simulink model "computed_torques_sim"  (R2019b)
settings: Solver=VariableStepAuto  StartTime=0.0  StopTime=10  MaxStep=1e-2  RelTol=1e-3
model workspace: external: MATLAB File /Users/simonlangbak/Desktop/CrustCrawlerModel/crustcrawler_DataFile.m (data not in the file)
undefined symbols (not defined in the file or in its folder): smiData, X, Y, Z
libraries: sm_lib x100, nesl_utility x10
(part 2 of 3)

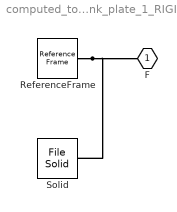
== system computed_torques_sim/Link 5/Link_plate_1_RIGID ==
  ReferenceFrame : sm_lib/Frames and Transforms/Reference Frame
  Solid : sm_lib/Body Elements/File Solid  ExtGeomFileName=Link-plate_Default_sldprt.STEP  UnitType=FromFile  ExtGeomFileUnits=m  StepReaderType=HEX  ExportEntireGeometry=off  InertiaType=Custom  Mass=smiData.Solid(7).mass  MassUnits=kg  CenterOfMass=smiData.Solid(7).CoM  CenterOfMassUnits=mm  MomentsOfInertia=smiData.Solid(7).MoI  MomentsOfInertiaUnits=kg*mm^2  ProductsOfInertia=smiData.Solid(7).PoI  ProductsOfInertiaUnits=kg*mm^2  BasedOnType=DensityFromFile  Density=1000  DensityUnits=kg/m^3  DoExposeReferenceFrame=on  SerializedFrames=<Frames/>  GraphicType=FromGeometry  MarkerShape=Sphere  MarkerSize=10  GraphicVisPropType=SimpleVisualProperties  GraphicDiffuseColor=smiData.Solid(7).color  GraphicSpecularColor=[0.5 0.5 0.5 1.0]  GraphicAmbientColor=[0.15 0.15 0.15 1.0]  GraphicEmissiveColor=[0.0 0.0 0.0 1.0]  GraphicShininess=75  GraphicOpacity=smiData.Solid(7).opacity
  F : PMIOPort  Side=Left
  connections:
  Solid/RConn1 -- ReferenceFrame/RConn1 -- F/RConn1

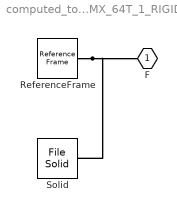
== system computed_torques_sim/Link 5/MX_64T_1_RIGID ==
  ReferenceFrame : sm_lib/Frames and Transforms/Reference Frame
  Solid : sm_lib/Body Elements/File Solid  ExtGeomFileName=MX-64T_Default_sldprt.STEP  UnitType=FromFile  ExtGeomFileUnits=m  StepReaderType=HEX  ExportEntireGeometry=off  InertiaType=Custom  Mass=smiData.Solid(14).mass  MassUnits=kg  CenterOfMass=smiData.Solid(14).CoM  CenterOfMassUnits=mm  MomentsOfInertia=smiData.Solid(14).MoI  MomentsOfInertiaUnits=kg*mm^2  ProductsOfInertia=smiData.Solid(14).PoI  ProductsOfInertiaUnits=kg*mm^2  BasedOnType=DensityFromFile  Density=1000  DensityUnits=kg/m^3  DoExposeReferenceFrame=on  SerializedFrames=<Frames/>  GraphicType=FromGeometry  MarkerShape=Sphere  MarkerSize=10  GraphicVisPropType=SimpleVisualProperties  GraphicDiffuseColor=smiData.Solid(14).color  GraphicSpecularColor=[0.5 0.5 0.5 1.0]  GraphicAmbientColor=[0.15 0.15 0.15 1.0]  GraphicEmissiveColor=[0.0 0.0 0.0 1.0]  GraphicShininess=75  GraphicOpacity=smiData.Solid(14).opacity
  F : PMIOPort  Side=Left
  connections:
  Solid/RConn1 -- ReferenceFrame/RConn1 -- F/RConn1

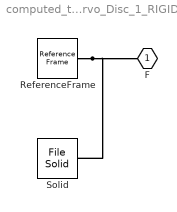
== system computed_torques_sim/Link 5/Servo_Disc_1_RIGID ==
  ReferenceFrame : sm_lib/Frames and Transforms/Reference Frame
  Solid : sm_lib/Body Elements/File Solid  ExtGeomFileName=Servo-Disc_Default_sldprt.STEP  UnitType=FromFile  ExtGeomFileUnits=m  StepReaderType=HEX  ExportEntireGeometry=off  InertiaType=Custom  Mass=smiData.Solid(3).mass  MassUnits=kg  CenterOfMass=smiData.Solid(3).CoM  CenterOfMassUnits=mm  MomentsOfInertia=smiData.Solid(3).MoI  MomentsOfInertiaUnits=kg*mm^2  ProductsOfInertia=smiData.Solid(3).PoI  ProductsOfInertiaUnits=kg*mm^2  BasedOnType=DensityFromFile  Density=1000  DensityUnits=kg/m^3  DoExposeReferenceFrame=on  SerializedFrames=<Frames/>  GraphicType=FromGeometry  MarkerShape=Sphere  MarkerSize=10  GraphicVisPropType=SimpleVisualProperties  GraphicDiffuseColor=smiData.Solid(3).color  GraphicSpecularColor=[0.5 0.5 0.5 1.0]  GraphicAmbientColor=[0.15 0.15 0.15 1.0]  GraphicEmissiveColor=[0.0 0.0 0.0 1.0]  GraphicShininess=75  GraphicOpacity=smiData.Solid(3).opacity
  F : PMIOPort  Side=Left
  connections:
  Solid/RConn1 -- ReferenceFrame/RConn1 -- F/RConn1

== system computed_torques_sim/Link 5/Servo_Disc_2_RIGID ==
  ReferenceFrame : sm_lib/Frames and Transforms/Reference Frame
  Solid : sm_lib/Body Elements/File Solid  ExtGeomFileName=Servo-Disc_Default_sldprt.STEP  UnitType=FromFile  ExtGeomFileUnits=m  StepReaderType=HEX  ExportEntireGeometry=off  InertiaType=Custom  Mass=smiData.Solid(3).mass  MassUnits=kg  CenterOfMass=smiData.Solid(3).CoM  CenterOfMassUnits=mm  MomentsOfInertia=smiData.Solid(3).MoI  MomentsOfInertiaUnits=kg*mm^2  ProductsOfInertia=smiData.Solid(3).PoI  ProductsOfInertiaUnits=kg*mm^2  BasedOnType=DensityFromFile  Density=1000  DensityUnits=kg/m^3  DoExposeReferenceFrame=on  SerializedFrames=<Frames/>  GraphicType=FromGeometry  MarkerShape=Sphere  MarkerSize=10  GraphicVisPropType=SimpleVisualProperties  GraphicDiffuseColor=smiData.Solid(3).color  GraphicSpecularColor=[0.5 0.5 0.5 1.0]  GraphicAmbientColor=[0.15 0.15 0.15 1.0]  GraphicEmissiveColor=[0.0 0.0 0.0 1.0]  GraphicShininess=75  GraphicOpacity=smiData.Solid(3).opacity
  F : PMIOPort  Side=Left
  connections:
  Solid/RConn1 -- ReferenceFrame/RConn1 -- F/RConn1

== system computed_torques_sim/Link 5/Servo_disc_link_MX_106T_1_RIGID ==
  ReferenceFrame : sm_lib/Frames and Transforms/Reference Frame
  Solid : sm_lib/Body Elements/File Solid  ExtGeomFileName=Servo-disc-link_MX-106T_Default_sldprt.STEP  UnitType=FromFile  ExtGeomFileUnits=m  StepReaderType=HEX  ExportEntireGeometry=off  InertiaType=Custom  Mass=smiData.Solid(16).mass  MassUnits=kg  CenterOfMass=smiData.Solid(16).CoM  CenterOfMassUnits=mm  MomentsOfInertia=smiData.Solid(16).MoI  MomentsOfInertiaUnits=kg*mm^2  ProductsOfInertia=smiData.Solid(16).PoI  ProductsOfInertiaUnits=kg*mm^2  BasedOnType=DensityFromFile  Density=1000  DensityUnits=kg/m^3  DoExposeReferenceFrame=on  SerializedFrames=<Frames/>  GraphicType=FromGeometry  MarkerShape=Sphere  MarkerSize=10  GraphicVisPropType=SimpleVisualProperties  GraphicDiffuseColor=smiData.Solid(16).color  GraphicSpecularColor=[0.5 0.5 0.5 1.0]  GraphicAmbientColor=[0.15 0.15 0.15 1.0]  GraphicEmissiveColor=[0.0 0.0 0.0 1.0]  GraphicShininess=75  GraphicOpacity=smiData.Solid(16).opacity
  F : PMIOPort  Side=Left
  connections:
  Solid/RConn1 -- ReferenceFrame/RConn1 -- F/RConn1

== system computed_torques_sim/Link 5/Servo_link_link_MX_64T_1_RIGID ==
  ReferenceFrame : sm_lib/Frames and Transforms/Reference Frame
  Solid : sm_lib/Body Elements/File Solid  ExtGeomFileName=Servo-link-link_MX-64T_Default_sldprt.STEP  UnitType=FromFile  ExtGeomFileUnits=m  StepReaderType=HEX  ExportEntireGeometry=off  InertiaType=Custom  Mass=smiData.Solid(13).mass  MassUnits=kg  CenterOfMass=smiData.Solid(13).CoM  CenterOfMassUnits=mm  MomentsOfInertia=smiData.Solid(13).MoI  MomentsOfInertiaUnits=kg*mm^2  ProductsOfInertia=smiData.Solid(13).PoI  ProductsOfInertiaUnits=kg*mm^2  BasedOnType=DensityFromFile  Density=1000  DensityUnits=kg/m^3  DoExposeReferenceFrame=on  SerializedFrames=<Frames/>  GraphicType=FromGeometry  MarkerShape=Sphere  MarkerSize=10  GraphicVisPropType=SimpleVisualProperties  GraphicDiffuseColor=smiData.Solid(13).color  GraphicSpecularColor=[0.5 0.5 0.5 1.0]  GraphicAmbientColor=[0.15 0.15 0.15 1.0]  GraphicEmissiveColor=[0.0 0.0 0.0 1.0]  GraphicShininess=75  GraphicOpacity=smiData.Solid(13).opacity
  F : PMIOPort  Side=Left
  connections:
  Solid/RConn1 -- ReferenceFrame/RConn1 -- F/RConn1

== system computed_torques_sim/Link 6/Finger_1_RIGID ==
  ReferenceFrame : sm_lib/Frames and Transforms/Reference Frame
  Solid : sm_lib/Body Elements/File Solid  ExtGeomFileName=Finger_Default_sldprt.STEP  UnitType=FromFile  ExtGeomFileUnits=m  StepReaderType=HEX  ExportEntireGeometry=off  InertiaType=Custom  Mass=smiData.Solid(4).mass  MassUnits=kg  CenterOfMass=smiData.Solid(4).CoM  CenterOfMassUnits=mm  MomentsOfInertia=smiData.Solid(4).MoI  MomentsOfInertiaUnits=kg*mm^2  ProductsOfInertia=smiData.Solid(4).PoI  ProductsOfInertiaUnits=kg*mm^2  BasedOnType=DensityFromFile  Density=1000  DensityUnits=kg/m^3  DoExposeReferenceFrame=on  SerializedFrames=<Frames/>  GraphicType=FromGeometry  MarkerShape=Sphere  MarkerSize=10  GraphicVisPropType=SimpleVisualProperties  GraphicDiffuseColor=smiData.Solid(4).color  GraphicSpecularColor=[0.5 0.5 0.5 1.0]  GraphicAmbientColor=[0.15 0.15 0.15 1.0]  GraphicEmissiveColor=[0.0 0.0 0.0 1.0]  GraphicShininess=75  GraphicOpacity=smiData.Solid(4).opacity
  F : PMIOPort  Side=Left
  connections:
  Solid/RConn1 -- ReferenceFrame/RConn1 -- F/RConn1

== system computed_torques_sim/Link 6/Finger_2_RIGID ==
  ReferenceFrame : sm_lib/Frames and Transforms/Reference Frame
  Solid : sm_lib/Body Elements/File Solid  ExtGeomFileName=Finger_Default_sldprt.STEP  UnitType=FromFile  ExtGeomFileUnits=m  StepReaderType=HEX  ExportEntireGeometry=off  InertiaType=Custom  Mass=smiData.Solid(4).mass  MassUnits=kg  CenterOfMass=smiData.Solid(4).CoM  CenterOfMassUnits=mm  MomentsOfInertia=smiData.Solid(4).MoI  MomentsOfInertiaUnits=kg*mm^2  ProductsOfInertia=smiData.Solid(4).PoI  ProductsOfInertiaUnits=kg*mm^2  BasedOnType=DensityFromFile  Density=1000  DensityUnits=kg/m^3  DoExposeReferenceFrame=on  SerializedFrames=<Frames/>  GraphicType=FromGeometry  MarkerShape=Sphere  MarkerSize=10  GraphicVisPropType=SimpleVisualProperties  GraphicDiffuseColor=smiData.Solid(4).color  GraphicSpecularColor=[0.5 0.5 0.5 1.0]  GraphicAmbientColor=[0.15 0.15 0.15 1.0]  GraphicEmissiveColor=[0.0 0.0 0.0 1.0]  GraphicShininess=75  GraphicOpacity=smiData.Solid(4).opacity
  F : PMIOPort  Side=Left
  connections:
  Solid/RConn1 -- ReferenceFrame/RConn1 -- F/RConn1

== system computed_torques_sim/Link 6/Link_2_1_RIGID ==
  ReferenceFrame : sm_lib/Frames and Transforms/Reference Frame
  Solid : sm_lib/Body Elements/File Solid  ExtGeomFileName=Link-2_Default_sldprt.STEP  UnitType=FromFile  ExtGeomFileUnits=m  StepReaderType=HEX  ExportEntireGeometry=off  InertiaType=Custom  Mass=smiData.Solid(8).mass  MassUnits=kg  CenterOfMass=smiData.Solid(8).CoM  CenterOfMassUnits=mm  MomentsOfInertia=smiData.Solid(8).MoI  MomentsOfInertiaUnits=kg*mm^2  ProductsOfInertia=smiData.Solid(8).PoI  ProductsOfInertiaUnits=kg*mm^2  BasedOnType=DensityFromFile  Density=1000  DensityUnits=kg/m^3  DoExposeReferenceFrame=on  SerializedFrames=<Frames/>  GraphicType=FromGeometry  MarkerShape=Sphere  MarkerSize=10  GraphicVisPropType=SimpleVisualProperties  GraphicDiffuseColor=smiData.Solid(8).color  GraphicSpecularColor=[0.5 0.5 0.5 1.0]  GraphicAmbientColor=[0.15 0.15 0.15 1.0]  GraphicEmissiveColor=[0.0 0.0 0.0 1.0]  GraphicShininess=75  GraphicOpacity=smiData.Solid(8).opacity
  F : PMIOPort  Side=Left
  connections:
  Solid/RConn1 -- ReferenceFrame/RConn1 -- F/RConn1

== system computed_torques_sim/Link 6/Link_plate_1_RIGID ==
  ReferenceFrame : sm_lib/Frames and Transforms/Reference Frame
  Solid : sm_lib/Body Elements/File Solid  ExtGeomFileName=Link-plate_Default_sldprt.STEP  UnitType=FromFile  ExtGeomFileUnits=m  StepReaderType=HEX  ExportEntireGeometry=off  InertiaType=Custom  Mass=smiData.Solid(7).mass  MassUnits=kg  CenterOfMass=smiData.Solid(7).CoM  CenterOfMassUnits=mm  MomentsOfInertia=smiData.Solid(7).MoI  MomentsOfInertiaUnits=kg*mm^2  ProductsOfInertia=smiData.Solid(7).PoI  ProductsOfInertiaUnits=kg*mm^2  BasedOnType=DensityFromFile  Density=1000  DensityUnits=kg/m^3  DoExposeReferenceFrame=on  SerializedFrames=<Frames/>  GraphicType=FromGeometry  MarkerShape=Sphere  MarkerSize=10  GraphicVisPropType=SimpleVisualProperties  GraphicDiffuseColor=smiData.Solid(7).color  GraphicSpecularColor=[0.5 0.5 0.5 1.0]  GraphicAmbientColor=[0.15 0.15 0.15 1.0]  GraphicEmissiveColor=[0.0 0.0 0.0 1.0]  GraphicShininess=75  GraphicOpacity=smiData.Solid(7).opacity
  F : PMIOPort  Side=Left
  connections:
  Solid/RConn1 -- ReferenceFrame/RConn1 -- F/RConn1

== system computed_torques_sim/Link 6/MX_28T_1_RIGID ==
  ReferenceFrame : sm_lib/Frames and Transforms/Reference Frame
  Solid : sm_lib/Body Elements/File Solid  ExtGeomFileName=MX-28T_Default_sldprt.STEP  UnitType=FromFile  ExtGeomFileUnits=m  StepReaderType=HEX  ExportEntireGeometry=off  InertiaType=Custom  Mass=smiData.Solid(5).mass  MassUnits=kg  CenterOfMass=smiData.Solid(5).CoM  CenterOfMassUnits=mm  MomentsOfInertia=smiData.Solid(5).MoI  MomentsOfInertiaUnits=kg*mm^2  ProductsOfInertia=smiData.Solid(5).PoI  ProductsOfInertiaUnits=kg*mm^2  BasedOnType=DensityFromFile  Density=1000  DensityUnits=kg/m^3  DoExposeReferenceFrame=on  SerializedFrames=<Frames/>  GraphicType=FromGeometry  MarkerShape=Sphere  MarkerSize=10  GraphicVisPropType=SimpleVisualProperties  GraphicDiffuseColor=smiData.Solid(5).color  GraphicSpecularColor=[0.5 0.5 0.5 1.0]  GraphicAmbientColor=[0.15 0.15 0.15 1.0]  GraphicEmissiveColor=[0.0 0.0 0.0 1.0]  GraphicShininess=75  GraphicOpacity=smiData.Solid(5).opacity
  F : PMIOPort  Side=Left
  connections:
  Solid/RConn1 -- ReferenceFrame/RConn1 -- F/RConn1

== system computed_torques_sim/Link 6/MX_28T_2_RIGID ==
  ReferenceFrame : sm_lib/Frames and Transforms/Reference Frame
  Solid : sm_lib/Body Elements/File Solid  ExtGeomFileName=MX-28T_Default_sldprt.STEP  UnitType=FromFile  ExtGeomFileUnits=m  StepReaderType=HEX  ExportEntireGeometry=off  InertiaType=Custom  Mass=smiData.Solid(5).mass  MassUnits=kg  CenterOfMass=smiData.Solid(5).CoM  CenterOfMassUnits=mm  MomentsOfInertia=smiData.Solid(5).MoI  MomentsOfInertiaUnits=kg*mm^2  ProductsOfInertia=smiData.Solid(5).PoI  ProductsOfInertiaUnits=kg*mm^2  BasedOnType=DensityFromFile  Density=1000  DensityUnits=kg/m^3  DoExposeReferenceFrame=on  SerializedFrames=<Frames/>  GraphicType=FromGeometry  MarkerShape=Sphere  MarkerSize=10  GraphicVisPropType=SimpleVisualProperties  GraphicDiffuseColor=smiData.Solid(5).color  GraphicSpecularColor=[0.5 0.5 0.5 1.0]  GraphicAmbientColor=[0.15 0.15 0.15 1.0]  GraphicEmissiveColor=[0.0 0.0 0.0 1.0]  GraphicShininess=75  GraphicOpacity=smiData.Solid(5).opacity
  F : PMIOPort  Side=Left
  connections:
  Solid/RConn1 -- ReferenceFrame/RConn1 -- F/RConn1

== system computed_torques_sim/Link 6/MX_28T_Link_1_RIGID ==
  ReferenceFrame : sm_lib/Frames and Transforms/Reference Frame
  Solid : sm_lib/Body Elements/File Solid  ExtGeomFileName=MX-28T-Link_Default_sldprt.STEP  UnitType=FromFile  ExtGeomFileUnits=m  StepReaderType=HEX  ExportEntireGeometry=off  InertiaType=Custom  Mass=smiData.Solid(9).mass  MassUnits=kg  CenterOfMass=smiData.Solid(9).CoM  CenterOfMassUnits=mm  MomentsOfInertia=smiData.Solid(9).MoI  MomentsOfInertiaUnits=kg*mm^2  ProductsOfInertia=smiData.Solid(9).PoI  ProductsOfInertiaUnits=kg*mm^2  BasedOnType=DensityFromFile  Density=1000  DensityUnits=kg/m^3  DoExposeReferenceFrame=on  SerializedFrames=<Frames/>  GraphicType=FromGeometry  MarkerShape=Sphere  MarkerSize=10  GraphicVisPropType=SimpleVisualProperties  GraphicDiffuseColor=smiData.Solid(9).color  GraphicSpecularColor=[0.5 0.5 0.5 1.0]  GraphicAmbientColor=[0.15 0.15 0.15 1.0]  GraphicEmissiveColor=[0.0 0.0 0.0 1.0]  GraphicShininess=75  GraphicOpacity=smiData.Solid(9).opacity
  F : PMIOPort  Side=Left
  connections:
  Solid/RConn1 -- ReferenceFrame/RConn1 -- F/RConn1

== system computed_torques_sim/Link 6/Servo_Disc_1_RIGID ==
  ReferenceFrame : sm_lib/Frames and Transforms/Reference Frame
  Solid : sm_lib/Body Elements/File Solid  ExtGeomFileName=Servo-Disc_Default_sldprt.STEP  UnitType=FromFile  ExtGeomFileUnits=m  StepReaderType=HEX  ExportEntireGeometry=off  InertiaType=Custom  Mass=smiData.Solid(3).mass  MassUnits=kg  CenterOfMass=smiData.Solid(3).CoM  CenterOfMassUnits=mm  MomentsOfInertia=smiData.Solid(3).MoI  MomentsOfInertiaUnits=kg*mm^2  ProductsOfInertia=smiData.Solid(3).PoI  ProductsOfInertiaUnits=kg*mm^2  BasedOnType=DensityFromFile  Density=1000  DensityUnits=kg/m^3  DoExposeReferenceFrame=on  SerializedFrames=<Frames/>  GraphicType=FromGeometry  MarkerShape=Sphere  MarkerSize=10  GraphicVisPropType=SimpleVisualProperties  GraphicDiffuseColor=smiData.Solid(3).color  GraphicSpecularColor=[0.5 0.5 0.5 1.0]  GraphicAmbientColor=[0.15 0.15 0.15 1.0]  GraphicEmissiveColor=[0.0 0.0 0.0 1.0]  GraphicShininess=75  GraphicOpacity=smiData.Solid(3).opacity
  F : PMIOPort  Side=Left
  connections:
  Solid/RConn1 -- ReferenceFrame/RConn1 -- F/RConn1

== system computed_torques_sim/Link 6/Servo_Disc_2_RIGID ==
  ReferenceFrame : sm_lib/Frames and Transforms/Reference Frame
  Solid : sm_lib/Body Elements/File Solid  ExtGeomFileName=Servo-Disc_Default_sldprt.STEP  UnitType=FromFile  ExtGeomFileUnits=m  StepReaderType=HEX  ExportEntireGeometry=off  InertiaType=Custom  Mass=smiData.Solid(3).mass  MassUnits=kg  CenterOfMass=smiData.Solid(3).CoM  CenterOfMassUnits=mm  MomentsOfInertia=smiData.Solid(3).MoI  MomentsOfInertiaUnits=kg*mm^2  ProductsOfInertia=smiData.Solid(3).PoI  ProductsOfInertiaUnits=kg*mm^2  BasedOnType=DensityFromFile  Density=1000  DensityUnits=kg/m^3  DoExposeReferenceFrame=on  SerializedFrames=<Frames/>  GraphicType=FromGeometry  MarkerShape=Sphere  MarkerSize=10  GraphicVisPropType=SimpleVisualProperties  GraphicDiffuseColor=smiData.Solid(3).color  GraphicSpecularColor=[0.5 0.5 0.5 1.0]  GraphicAmbientColor=[0.15 0.15 0.15 1.0]  GraphicEmissiveColor=[0.0 0.0 0.0 1.0]  GraphicShininess=75  GraphicOpacity=smiData.Solid(3).opacity
  F : PMIOPort  Side=Left
  connections:
  Solid/RConn1 -- ReferenceFrame/RConn1 -- F/RConn1

== system computed_torques_sim/Link 6/Servo_Disc_3_RIGID ==
  ReferenceFrame : sm_lib/Frames and Transforms/Reference Frame
  Solid : sm_lib/Body Elements/File Solid  ExtGeomFileName=Servo-Disc_Default_sldprt.STEP  UnitType=FromFile  ExtGeomFileUnits=m  StepReaderType=HEX  ExportEntireGeometry=off  InertiaType=Custom  Mass=smiData.Solid(3).mass  MassUnits=kg  CenterOfMass=smiData.Solid(3).CoM  CenterOfMassUnits=mm  MomentsOfInertia=smiData.Solid(3).MoI  MomentsOfInertiaUnits=kg*mm^2  ProductsOfInertia=smiData.Solid(3).PoI  ProductsOfInertiaUnits=kg*mm^2  BasedOnType=DensityFromFile  Density=1000  DensityUnits=kg/m^3  DoExposeReferenceFrame=on  SerializedFrames=<Frames/>  GraphicType=FromGeometry  MarkerShape=Sphere  MarkerSize=10  GraphicVisPropType=SimpleVisualProperties  GraphicDiffuseColor=smiData.Solid(3).color  GraphicSpecularColor=[0.5 0.5 0.5 1.0]  GraphicAmbientColor=[0.15 0.15 0.15 1.0]  GraphicEmissiveColor=[0.0 0.0 0.0 1.0]  GraphicShininess=75  GraphicOpacity=smiData.Solid(3).opacity
  F : PMIOPort  Side=Left
  connections:
  Solid/RConn1 -- ReferenceFrame/RConn1 -- F/RConn1

== system computed_torques_sim/Link 6/Servo_Disc_4_RIGID ==
  ReferenceFrame : sm_lib/Frames and Transforms/Reference Frame
  Solid : sm_lib/Body Elements/File Solid  ExtGeomFileName=Servo-Disc_Default_sldprt.STEP  UnitType=FromFile  ExtGeomFileUnits=m  StepReaderType=HEX  ExportEntireGeometry=off  InertiaType=Custom  Mass=smiData.Solid(3).mass  MassUnits=kg  CenterOfMass=smiData.Solid(3).CoM  CenterOfMassUnits=mm  MomentsOfInertia=smiData.Solid(3).MoI  MomentsOfInertiaUnits=kg*mm^2  ProductsOfInertia=smiData.Solid(3).PoI  ProductsOfInertiaUnits=kg*mm^2  BasedOnType=DensityFromFile  Density=1000  DensityUnits=kg/m^3  DoExposeReferenceFrame=on  SerializedFrames=<Frames/>  GraphicType=FromGeometry  MarkerShape=Sphere  MarkerSize=10  GraphicVisPropType=SimpleVisualProperties  GraphicDiffuseColor=smiData.Solid(3).color  GraphicSpecularColor=[0.5 0.5 0.5 1.0]  GraphicAmbientColor=[0.15 0.15 0.15 1.0]  GraphicEmissiveColor=[0.0 0.0 0.0 1.0]  GraphicShininess=75  GraphicOpacity=smiData.Solid(3).opacity
  F : PMIOPort  Side=Left
  connections:
  Solid/RConn1 -- ReferenceFrame/RConn1 -- F/RConn1

== system computed_torques_sim/Link 6/Servo_Disc_5_RIGID ==
  ReferenceFrame : sm_lib/Frames and Transforms/Reference Frame
  Solid : sm_lib/Body Elements/File Solid  ExtGeomFileName=Servo-Disc_Default_sldprt.STEP  UnitType=FromFile  ExtGeomFileUnits=m  StepReaderType=HEX  ExportEntireGeometry=off  InertiaType=Custom  Mass=smiData.Solid(3).mass  MassUnits=kg  CenterOfMass=smiData.Solid(3).CoM  CenterOfMassUnits=mm  MomentsOfInertia=smiData.Solid(3).MoI  MomentsOfInertiaUnits=kg*mm^2  ProductsOfInertia=smiData.Solid(3).PoI  ProductsOfInertiaUnits=kg*mm^2  BasedOnType=DensityFromFile  Density=1000  DensityUnits=kg/m^3  DoExposeReferenceFrame=on  SerializedFrames=<Frames/>  GraphicType=FromGeometry  MarkerShape=Sphere  MarkerSize=10  GraphicVisPropType=SimpleVisualProperties  GraphicDiffuseColor=smiData.Solid(3).color  GraphicSpecularColor=[0.5 0.5 0.5 1.0]  GraphicAmbientColor=[0.15 0.15 0.15 1.0]  GraphicEmissiveColor=[0.0 0.0 0.0 1.0]  GraphicShininess=75  GraphicOpacity=smiData.Solid(3).opacity
  F : PMIOPort  Side=Left
  connections:
  Solid/RConn1 -- ReferenceFrame/RConn1 -- F/RConn1

== system computed_torques_sim/Link 6/Servo_Disc_6_RIGID ==
  ReferenceFrame : sm_lib/Frames and Transforms/Reference Frame
  Solid : sm_lib/Body Elements/File Solid  ExtGeomFileName=Servo-Disc_Default_sldprt.STEP  UnitType=FromFile  ExtGeomFileUnits=m  StepReaderType=HEX  ExportEntireGeometry=off  InertiaType=Custom  Mass=smiData.Solid(3).mass  MassUnits=kg  CenterOfMass=smiData.Solid(3).CoM  CenterOfMassUnits=mm  MomentsOfInertia=smiData.Solid(3).MoI  MomentsOfInertiaUnits=kg*mm^2  ProductsOfInertia=smiData.Solid(3).PoI  ProductsOfInertiaUnits=kg*mm^2  BasedOnType=DensityFromFile  Density=1000  DensityUnits=kg/m^3  DoExposeReferenceFrame=on  SerializedFrames=<Frames/>  GraphicType=FromGeometry  MarkerShape=Sphere  MarkerSize=10  GraphicVisPropType=SimpleVisualProperties  GraphicDiffuseColor=smiData.Solid(3).color  GraphicSpecularColor=[0.5 0.5 0.5 1.0]  GraphicAmbientColor=[0.15 0.15 0.15 1.0]  GraphicEmissiveColor=[0.0 0.0 0.0 1.0]  GraphicShininess=75  GraphicOpacity=smiData.Solid(3).opacity
  F : PMIOPort  Side=Left
  connections:
  Solid/RConn1 -- ReferenceFrame/RConn1 -- F/RConn1

== system computed_torques_sim/Link 6/Servo_disc_link_MX_28T_1_RIGID ==
  ReferenceFrame : sm_lib/Frames and Transforms/Reference Frame
  Solid : sm_lib/Body Elements/File Solid  ExtGeomFileName=Servo-disc-link_MX-28T_Default_sldprt.STEP  UnitType=FromFile  ExtGeomFileUnits=m  StepReaderType=HEX  ExportEntireGeometry=off  InertiaType=Custom  Mass=smiData.Solid(10).mass  MassUnits=kg  CenterOfMass=smiData.Solid(10).CoM  CenterOfMassUnits=mm  MomentsOfInertia=smiData.Solid(10).MoI  MomentsOfInertiaUnits=kg*mm^2  ProductsOfInertia=smiData.Solid(10).PoI  ProductsOfInertiaUnits=kg*mm^2  BasedOnType=DensityFromFile  Density=1000  DensityUnits=kg/m^3  DoExposeReferenceFrame=on  SerializedFrames=<Frames/>  GraphicType=FromGeometry  MarkerShape=Sphere  MarkerSize=10  GraphicVisPropType=SimpleVisualProperties  GraphicDiffuseColor=smiData.Solid(10).color  GraphicSpecularColor=[0.5 0.5 0.5 1.0]  GraphicAmbientColor=[0.15 0.15 0.15 1.0]  GraphicEmissiveColor=[0.0 0.0 0.0 1.0]  GraphicShininess=75  GraphicOpacity=smiData.Solid(10).opacity
  F : PMIOPort  Side=Left
  connections:
  Solid/RConn1 -- ReferenceFrame/RConn1 -- F/RConn1

== system computed_torques_sim/Link 6/Servo_disc_link_MX_28T_2_RIGID ==
  ReferenceFrame : sm_lib/Frames and Transforms/Reference Frame
  Solid : sm_lib/Body Elements/File Solid  ExtGeomFileName=Servo-disc-link_MX-28T_Default_sldprt.STEP  UnitType=FromFile  ExtGeomFileUnits=m  StepReaderType=HEX  ExportEntireGeometry=off  InertiaType=Custom  Mass=smiData.Solid(10).mass  MassUnits=kg  CenterOfMass=smiData.Solid(10).CoM  CenterOfMassUnits=mm  MomentsOfInertia=smiData.Solid(10).MoI  MomentsOfInertiaUnits=kg*mm^2  ProductsOfInertia=smiData.Solid(10).PoI  ProductsOfInertiaUnits=kg*mm^2  BasedOnType=DensityFromFile  Density=1000  DensityUnits=kg/m^3  DoExposeReferenceFrame=on  SerializedFrames=<Frames/>  GraphicType=FromGeometry  MarkerShape=Sphere  MarkerSize=10  GraphicVisPropType=SimpleVisualProperties  GraphicDiffuseColor=smiData.Solid(10).color  GraphicSpecularColor=[0.5 0.5 0.5 1.0]  GraphicAmbientColor=[0.15 0.15 0.15 1.0]  GraphicEmissiveColor=[0.0 0.0 0.0 1.0]  GraphicShininess=75  GraphicOpacity=smiData.Solid(10).opacity
  F : PMIOPort  Side=Left
  connections:
  Solid/RConn1 -- ReferenceFrame/RConn1 -- F/RConn1

== system computed_torques_sim/Link 6/Servo_disc_link_MX_64T_1_RIGID ==
  ReferenceFrame : sm_lib/Frames and Transforms/Reference Frame
  Solid : sm_lib/Body Elements/File Solid  ExtGeomFileName=Servo-disc-link_MX-64T_Default_sldprt.STEP  UnitType=FromFile  ExtGeomFileUnits=m  StepReaderType=HEX  ExportEntireGeometry=off  InertiaType=Custom  Mass=smiData.Solid(2).mass  MassUnits=kg  CenterOfMass=smiData.Solid(2).CoM  CenterOfMassUnits=mm  MomentsOfInertia=smiData.Solid(2).MoI  MomentsOfInertiaUnits=kg*mm^2  ProductsOfInertia=smiData.Solid(2).PoI  ProductsOfInertiaUnits=kg*mm^2  BasedOnType=DensityFromFile  Density=1000  DensityUnits=kg/m^3  DoExposeReferenceFrame=on  SerializedFrames=<Frames/>  GraphicType=FromGeometry  MarkerShape=Sphere  MarkerSize=10  GraphicVisPropType=SimpleVisualProperties  GraphicDiffuseColor=smiData.Solid(2).color  GraphicSpecularColor=[0.5 0.5 0.5 1.0]  GraphicAmbientColor=[0.15 0.15 0.15 1.0]  GraphicEmissiveColor=[0.0 0.0 0.0 1.0]  GraphicShininess=75  GraphicOpacity=smiData.Solid(2).opacity
  F : PMIOPort  Side=Left
  connections:
  Solid/RConn1 -- ReferenceFrame/RConn1 -- F/RConn1

== system computed_torques_sim/Link 6/Servo_link_link_MX_28T_1_RIGID ==
  ReferenceFrame : sm_lib/Frames and Transforms/Reference Frame
  Solid : sm_lib/Body Elements/File Solid  ExtGeomFileName=Servo-link-link_MX-28T_Default_sldprt.STEP  UnitType=FromFile  ExtGeomFileUnits=m  StepReaderType=HEX  ExportEntireGeometry=off  InertiaType=Custom  Mass=smiData.Solid(6).mass  MassUnits=kg  CenterOfMass=smiData.Solid(6).CoM  CenterOfMassUnits=mm  MomentsOfInertia=smiData.Solid(6).MoI  MomentsOfInertiaUnits=kg*mm^2  ProductsOfInertia=smiData.Solid(6).PoI  ProductsOfInertiaUnits=kg*mm^2  BasedOnType=DensityFromFile  Density=1000  DensityUnits=kg/m^3  DoExposeReferenceFrame=on  SerializedFrames=<Frames/>  GraphicType=FromGeometry  MarkerShape=Sphere  MarkerSize=10  GraphicVisPropType=SimpleVisualProperties  GraphicDiffuseColor=smiData.Solid(6).color  GraphicSpecularColor=[0.5 0.5 0.5 1.0]  GraphicAmbientColor=[0.15 0.15 0.15 1.0]  GraphicEmissiveColor=[0.0 0.0 0.0 1.0]  GraphicShininess=75  GraphicOpacity=smiData.Solid(6).opacity
  F : PMIOPort  Side=Left
  connections:
  Solid/RConn1 -- ReferenceFrame/RConn1 -- F/RConn1

== matlab function computed_torques_sim/Mass matrix ==
  data: theta1 input; M output; theta2 input; theta3 input
function M = mass_matrix(theta1, theta2, theta3)
q1= theta1;
q2=theta2;
q3=theta3;

Mass_m = [(1615035341814929905506560793992835710915519260448843256958658427314649*sin(2*q2 + q3))/13164036458569648337239753460458804039861886925068638906788872192000000000 - (457511997578021908713815184616433992939798263502173106608732750872146873*sin(2*q2))/32910091146424120843099383651147010099654717312671597266972180480000000000000 + (255908045475753844730133796297136773933654114624346529772767709464560837*sin(2*q2 + 2*q3))/3291009114642412084309938365114701009965471731267159726697218048000000000000 + (4828675901527893559178853*sin(q2 + q3))/633825300114114700748351602688000000000000000 + (73416068380051054984947309*sin(q2))/5070602400912917605986812821504000000000000000 + (40375883545373247637664019849821195543519635458506643231420221127225807*sin(q3))/329100911464241208430993836511470100996547173126715972669721804800000000000 - (731837300205207575605568155447709406028814655043735155356881565467998260091*sin(q2 + q3)^2)/131640364585696483372397534604588040398618869250686389067888721920000000000000 - (548849207189820860977438276832289608921204175355689439784044105294748774809*sin(q2)^2)/26328072917139296674479506920917608079723773850137277813577744384000000000000 - (72179656430344175007639370869987503695532053101598302484075426636139313*sin(q2 + q3/2)^2)/4113761393303015105387422956393376262456839664083949658371522560000000000 - (6186005764032386164041*sin(q2/2)^2)/633825300114114700748351602688000000000000000 - (1804491410758604375190984271749701123906531400107104593650396036532168759*sin(q3/2)^2)/102844034832575377634685573909834406561420991602098741459288064000000000000 + (108042662168438237985069*sin(q2/2 + q3/2)^2)/507060240091291760598681282150400000000000000 + 144652079847309965235720252633995975024744360907149566056558400284822875644659/3291009114642412084309938365114701009965471731267159726697218048000000000000000 (24678615572571482867467662723121*cos(3*q2))/1316403645856964833723975346045880403986188692506863890678887219200000000000 - (13164036458569648337239753460458828718477459496551506374451595313*sin(q2 + 2*q3))/26328072917139296674479506920917608079723773850137277813577744384000000000 - (101851798816724308024107115849748350880707213226788621691314151818815458137090251*cos(q2 + 2*q3))/4074071952668972172536891376818756322102936787331872501272280898708762599526673412366794752 + (24678615572571482867467662723121*sin(3*q2))/26328072917139296674479506920917608079723773850137277813577744384000000000 + (190941539571362125253113645164323100745595889867*cos(3*q2 + 2*q3))/4074071952668972172536891376818756322102936787331872501272280898708762599526673412366794752 + (24678615572571482867467662723121*sin(3*q2 + 2*q3))/26328072917139296674479506920917608079723773850137277813577744384000000000 - (21748779*cos(q2 + q3))/25000000000000 + (972003123*sin(q2 + q3))/15625000000000 + (32780418805288980521239894429846520292708990430992695097595195969962079*cos(q2))/822752278660603021077484591278675252491367932816789931674304512000000000000000 + (1361934228636072542332497*cos(q3))/1267650600228229401496703205376000000000000 + (48636014041917239509817246664812018588988042524514863263996327308385782087*sin(q2))/411376139330301510538742295639337626245683966408394965837152256000000000000000 + (30473571380841554303481*sin(q3))/2028240960365167042394725128601600000000000 + 1311892280924518464958274969/811296384146066816957890051440640000000000000 (190941539571362125253113645164323100745595889867*cos(3*q2 + 3*q3))/4074071952668972172536891376818756322102936787331872501272280898708762599526673412366794752 + (24678615572571482867467662723121*sin(3*q2 + 3*q3))/26328072917139296674479506920917608079723773850137277813577744384000000000 - (21632843643718816021471397072348521912991774124847858673204606804210679038703548492923897949123*cos(q2 + q3))/24866161820489332107769112407341042005022807539867385872023198844657974850626668776652800000000000000 + (25590763409961451442862325755484209409982814949374534396229078538366945607*sin(q2 + q3))/411376139330301510538742295639337626245683966408394965837152256000000000000000 + (1361934228636072542332497*cos(q3))/2535301200456458802993406410752000000000000 + (30473571380841554303481*sin(q3))/4056481920730334084789450257203200000000000 + 13814199891355225887065509029/40564819207303340847894502572032000000000000000;
      (24678615572571482867467662723121*cos(3*q2))/1316403645856964833723975346045880403986188692506863890678887219200000000000 - (13164036458569648337239753460458828718477459496551506374451595313*sin(q2 + 2*q3))/26328072917139296674479506920917608079723773850137277813577744384000000000 - (101851798816724308024107115849748350880707213226788621691314151818815458137090251*cos(q2 + 2*q3))/4074071952668972172536891376818756322102936787331872501272280898708762599526673412366794752 + (24678615572571482867467662723121*sin(3*q2))/26328072917139296674479506920917608079723773850137277813577744384000000000 + (190941539571362125253113645164323100745595889867*cos(3*q2 + 2*q3))/4074071952668972172536891376818756322102936787331872501272280898708762599526673412366794752 + (24678615572571482867467662723121*sin(3*q2 + 2*q3))/26328072917139296674479506920917608079723773850137277813577744384000000000 - (21748779*cos(q2 + q3))/25000000000000 + (972003123*sin(q2 + q3))/15625000000000 + (32780418805288980521239894429846520292708990430992695097595195969962079*cos(q2))/822752278660603021077484591278675252491367932816789931674304512000000000000000 + (1361934228636072542332497*cos(q3))/1267650600228229401496703205376000000000000 + (48636014041917239509817246664812018588988042524514863263996327308385782087*sin(q2))/411376139330301510538742295639337626245683966408394965837152256000000000000000 + (30473571380841554303481*sin(q3))/2028240960365167042394725128601600000000000 + 1311892280924518464958274969/811296384146066816957890051440640000000000000 (151385315826973642780903726880222179791*sin(2*q2 + q3))/329100911464241208430993836511470100996547173126715972669721804800000000000 - (141124381657242464255308204087741708981790336338868593870928986372549559319728027525029551289217810562711*sin(2*q2))/2707685248164858261307045101702230179137145581421695874189921465443966120903931272499975005961073806735733604454495675614232576000000000000000 - (173291855882550928723650886508943381205167605922343745470406444080806175046695813871987190748514248698142627759379988450723567969*sin(2*q3))/346583711765101857447301773017885462929554634421977071896309947576827663475703202879996800763017447262173901370175446478621769728000000000 - (609034066578767699168763939638324732237239140958410949107980641*sin(4*q2))/346583711765101857447301773017885462929554634421977071896309947576827663475703202879996800763017447262173901370175446478621769728000000000 + (157888437344326403338797001820296661107270341343067227696504764466979317853222477129365328258806685551893*sin(2*q2 + 2*q3))/541537049632971652261409020340446035827429116284339174837984293088793224180786254499995001192214761347146720890899135122846515200000000000000 - (609034066578767699168763939638324732237239140958410949107980641*sin(4*q2 + 2*q3))/346583711765101857447301773017885462929554634421977071896309947576827663475703202879996800763017447262173901370175446478621769728000000000 + (80751767090746495275328039699642239701723443943370505559113562032271823*sin(q3))/329100911464241208430993836511470100996547173126715972669721804800000000000 - (8528939412261526414013495183883659144516921448299527172658426609424218670365243171019180172363562838514818030842315720105453541791*sin(q2 + q3)^2)/409173825987017733751648712103449894027080255755383098685411421012016724550584319360408761540738019643860835515945008876152157068235674131666065948672000000000000000 - (6396369187265599931466306206240927025452851013153542767551139149872066624680215503864376155768695238461799489217022009354501927539*sin(q2)^2)/81834765197403546750329742420689978805416051151076619737082284202403344910116863872081752308147603928772167103189001775230431413647134826333213189734400000000000000 + (1340780792994259758804992907016991404613268737920347276692458624772422856441187592116416438926026948482165122837780450213256421346417542809593563*sin(q3)^2)/26815615859885194199148049996411692254958731641184786755447122887443528060147093953603748596333806855380063716372972101707507765623893139892867298012168192 + (4712172851916591368075437063825668450117988598500996060499981207992026430514907*sin(2*q2 + q3)^2)/26815615859885194199148049996411692254958731641184786755447122887443528060147093953603748596333806855380063716372972101707507765623893139892867298012168192 - (6765759115036283573515774255185314342967*sin(q2 + q3/2)^2)/102844034832575377634685573909834406561420991602098741459288064000000000000 + (609034066578767699168763939638324732237239140958410949107980641*sin(2*q2)^2)/8664592794127546436182544325447136573238865860549426797407748689420691586892580071999920019075436181554347534254386161965544243200000000000 - (3608982821517208750381968543499395482053947763930635671526536887749994551*sin(q3/2)^2)/102844034832575377634685573909834406561420991602098741459288064000000000000 + 144653147798638312962142186726283544288868940043546260848924718907717985756987/3291009114642412084309938365114701009965471731267159726697218048000000000000000 (215345230439164413868879837916658197201957296168653475451074726596863972314148369725284003754939957667875566640224098471920888353*cos(2*q2 + q3))/13093562431584567480052758787310396608866568184172259157933165472384535185618698219533080369303616628603546736510240284036869026183541572213314110357504000000000000 + (1992849938593240455708175754552602502608601647638750571957635744944730656008201327588393193071252568697*sin(2*q2 + q3))/8664592794127546436182544325447136573238865860549426797407748689420691586892580071999920019075436181554347534254386161965544243200000000000 + (68598760010690564171920024416429451723759869*cos(2*q2 + 2*q3))/6582018229284824168619876730229402019930943462534319453394436096000000000000000 + (2513561388372830240079175525293217039494524600214065313681558420906869044421417766570763039836190421514001393371*cos(2*q2 + 3*q3))/53631231719770388398296099992823384509917463282369573510894245774887056120294187907207497192667613710760127432745944203415015531247786279785734596024336384 - (4712172851916591368075437063825668450117988598500996060499981207992026430514907*cos(4*q2 + 3*q3))/53631231719770388398296099992823384509917463282369573510894245774887056120294187907207497192667613710760127432745944203415015531247786279785734596024336384 + (23987691407855914487919563268384296306883*sin(2*q2 + 2*q3))/82275227866060302107748459127867525249136793281678993167430451200000000000000 + (324870195144355677604761125735146500688687711490065578777153321924899646458107625338080260331873*sin(2*q2 + 3*q3))/346583711765101857447301773017885462929554634421977071896309947576827663475703202879996800763017447262173901370175446478621769728000000000 - (609034066578767699168763939638324732237239140958410949107980641*sin(4*q2 + 3*q3))/346583711765101857447301773017885462929554634421977071896309947576827663475703202879996800763017447262173901370175446478621769728000000000 + (114869184822561496165330768925189088253207077043060138712725207712562956161635106029426841109235611779388119865989562898864555314957084222009354206048520078792159*cos(q3))/13093562431584567480052758787310396608866568184172259157933165472384535185618698219533080369303616628603546736510240284036869026183541572213314110357504000000000000 + (1063014873780114504319340555963937907542457727596866615041223323514049029958436959584913945993225298443507443540144666382960617660646791*sin(q3))/8664592794127546436182544325447136573238865860549426797407748689420691586892580071999920019075436181554347534254386161965544243200000000000 + 36606180425345558941409345436650155999799196483621368788458943511388077925507/6582018229284824168619876730229402019930943462534319453394436096000000000000000;
     (190941539571362125253113645164323100745595889867*cos(3*q2 + 3*q3))/4074071952668972172536891376818756322102936787331872501272280898708762599526673412366794752 + (24678615572571482867467662723121*sin(3*q2 + 3*q3))/26328072917139296674479506920917608079723773850137277813577744384000000000 - (21632843643718816021471397072348521912991774124847858673204606804210679038703548492923897949123*cos(q2 + q3))/24866161820489332107769112407341042005022807539867385872023198844657974850626668776652800000000000000 + (25590763409961451442862325755484209409982814949374534396229078538366945607*sin(q2 + q3))/411376139330301510538742295639337626245683966408394965837152256000000000000000 + (1361934228636072542332497*cos(q3))/2535301200456458802993406410752000000000000 + (30473571380841554303481*sin(q3))/4056481920730334084789450257203200000000000 + 13814199891355225887065509029/40564819207303340847894502572032000000000000000 (215345230439164413868879837916658197201957296168653475451074726596863972314148369725284003754939957667875566640224098471920888353*cos(2*q2 + q3))/13093562431584567480052758787310396608866568184172259157933165472384535185618698219533080369303616628603546736510240284036869026183541572213314110357504000000000000 + (1992849938593240455708175754552602502608601647638750571957635744944730656008201327588393193071252568697*sin(2*q2 + q3))/8664592794127546436182544325447136573238865860549426797407748689420691586892580071999920019075436181554347534254386161965544243200000000000 + (68598760010690564171920024416429451723759869*cos(2*q2 + 2*q3))/6582018229284824168619876730229402019930943462534319453394436096000000000000000 + (2513561388372830240079175525293217039494524600214065313681558420906869044421417766570763039836190421514001393371*cos(2*q2 + 3*q3))/53631231719770388398296099992823384509917463282369573510894245774887056120294187907207497192667613710760127432745944203415015531247786279785734596024336384 - (4712172851916591368075437063825668450117988598500996060499981207992026430514907*cos(4*q2 + 3*q3))/53631231719770388398296099992823384509917463282369573510894245774887056120294187907207497192667613710760127432745944203415015531247786279785734596024336384 + (23987691407855914487919563268384296306883*sin(2*q2 + 2*q3))/82275227866060302107748459127867525249136793281678993167430451200000000000000 + (324870195144355677604761125735146500688687711490065578777153321924899646458107625338080260331873*sin(2*q2 + 3*q3))/346583711765101857447301773017885462929554634421977071896309947576827663475703202879996800763017447262173901370175446478621769728000000000 - (609034066578767699168763939638324732237239140958410949107980641*sin(4*q2 + 3*q3))/346583711765101857447301773017885462929554634421977071896309947576827663475703202879996800763017447262173901370175446478621769728000000000 + (114869184822561496165330768925189088253207077043060138712725207712562956161635106029426841109235611779388119865989562898864555314957084222009354206048520078792159*cos(q3))/13093562431584567480052758787310396608866568184172259157933165472384535185618698219533080369303616628603546736510240284036869026183541572213314110357504000000000000 + (1063014873780114504319340555963937907542457727596866615041223323514049029958436959584913945993225298443507443540144666382960617660646791*sin(q3))/8664592794127546436182544325447136573238865860549426797407748689420691586892580071999920019075436181554347534254386161965544243200000000000 + 36606180425345558941409345436650155999799196483621368788458943511388077925507/6582018229284824168619876730229402019930943462534319453394436096000000000000000 (157888437344326403338797001820296661107270341343067227696504764466979317853222477129365328258806685551893*sin(2*q2 + 2*q3))/541537049632971652261409020340446035827429116284339174837984293088793224180786254499995001192214761347146720890899135122846515200000000000000 - (609034066578767699168763939638324732237239140958410949107980641*sin(4*q2 + 4*q3))/346583711765101857447301773017885462929554634421977071896309947576827663475703202879996800763017447262173901370175446478621769728000000000 - (4264469698459982602841618226894267204760103088736332403708778928777858112112212985305812264003222692386865358946912469351432825583*sin(q2 + q3)^2)/204586912993508866875824356051724947013540127877691549342705710506008362275292159680204380770369009821930417757972504438076078534117837065833032974336000000000000000 + (4712172851916591368075437063825668450117988598500996060499981207992026430514907*sin(2*q2 + 2*q3)^2)/26815615859885194199148049996411692254958731641184786755447122887443528060147093953603748596333806855380063716372972101707507765623893139892867298012168192 + 285985783544571830904006630947232653909017096215507467262082249537810950667/51422017416287688817342786954917203280710495801049370729644032000000000000000];

M = Mass_m;
